simulink model "modal_closed_loop_control_Q27"  (R2025b)
settings: Solver=VariableStepAuto  StartTime=0.0  StopTime=200  RelTol=1e-3
undefined symbols (not defined in the file or in its folder): alpha, Den, eta_0, H, Jr, Js, K, Num, omega, sigma_m_square, taue, taum, Tc_max, theta_ref_FV, Torque_disturbance, xi
libraries: simulink_extras x2
settings Model: Creator=flori  LastModifiedBy=flori
settings DebuggingCC: AlgebraicLoopMsg=none

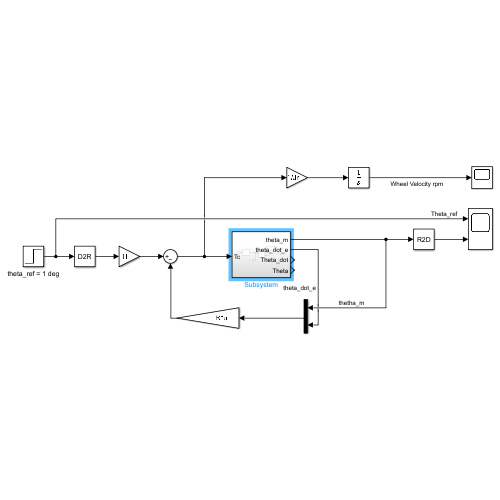
[thumbnail: Simulink's stored preview of the top-level diagram]
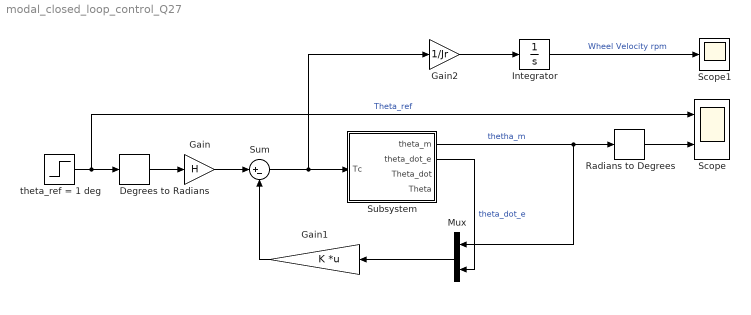
== system modal_closed_loop_control_Q27 ==
  Degrees to Radians : simulink_extras/Transformations/Degrees to Radians
  Gain : Gain  Gain=H
  Gain1 : Gain  Gain=K  Multiplication=Matrix(K*u)
  Gain2 : Gain  Gain=1/Jr
  Integrator : Integrator
  Mux : Mux  Inputs=2
  Radians to Degrees : simulink_extras/Transformations/Radians to Degrees
  Scope : Scope  NumInputPorts=2
      settings: ActiveDisplayYMinimum=-1.2780559634546143  ActiveDisplayYMaximum=11.460603856286715
  Scope1 : Scope
      settings: ActiveDisplayYMinimum=-162.46244989457873  ActiveDisplayYMaximum=1462.1620490512087
  Subsystem : Subsystem
  Sum : Sum  Inputs=|+-
  theta_ref = 1 deg : Step  Time=0  After=theta_ref_FV  SampleTime=0
  wires:
  Gain/1 -> Sum/1
  Mux/1 -> Gain1/1
  Subsystem/1(theta_m) -> Radians to Degrees/1, Mux/1  "thetha_m"
  Subsystem/2(theta_dot_e) -> Mux/2  "theta_dot_e"
  Gain2/1 -> Integrator/1
  Integrator/1 -> Scope1/1  "Wheel Velocity rpm"
  theta_ref = 1 deg/1 -> Scope/1, Degrees to Radians/1  "Theta_ref"
  Degrees to Radians/1 -> Gain/1
  Radians to Degrees/1 -> Scope/2
  Gain1/1 -> Sum/2
  Sum/1 -> Gain2/1, Subsystem/1(Tc)

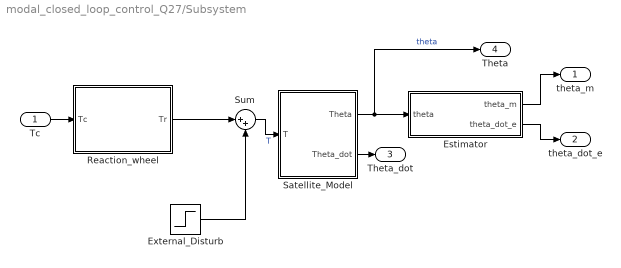
== system modal_closed_loop_control_Q27/Subsystem ==
  Tc : Inport
  Estimator : Subsystem
  External_Disturb : Step  Time=100  After=Torque_disturbance  SampleTime=0
  Reaction_wheel : Subsystem
  Satellite_Model : Subsystem
  Sum : Sum  Inputs=|++
  theta_m : Outport
  theta_dot_e : Outport  Port=2
  Theta_dot : Outport  Port=3
  Theta : Outport  Port=4
  wires:
  Satellite_Model/1(Theta) -> Theta/1, Estimator/1(theta)  "theta"
  Sum/1 -> Satellite_Model/1(T)  "T"
  Reaction_wheel/1(Tr) -> Sum/1
  Estimator/2(theta_dot_e) -> theta_dot_e/1
  Estimator/1(theta_m) -> theta_m/1
  Satellite_Model/2(Theta_dot) -> Theta_dot/1
  Tc/1 -> Reaction_wheel/1(Tc)
  External_Disturb/1 -> Sum/2

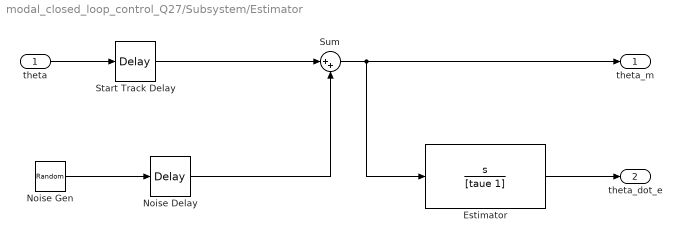
== system modal_closed_loop_control_Q27/Subsystem/Estimator ==
  theta : Inport
  Estimator : TransferFcn  Numerator=[1 0]  Denominator=[taue 1]
  Noise Delay : TransportDelay  DelayTime=160
  Noise Gen : RandomNumber  Variance=sigma_m_square  SampleTime=0.01
  Start Track Delay : TransportDelay  DelayTime=taum
  Sum : Sum  Inputs=|++
  theta_m : Outport
  theta_dot_e : Outport  Port=2
  wires:
  Start Track Delay/1 -> Sum/1
  Sum/1 -> theta_m/1, Estimator/1
  theta/1 -> Start Track Delay/1
  Estimator/1 -> theta_dot_e/1
  Noise Gen/1 -> Noise Delay/1
  Noise Delay/1 -> Sum/2

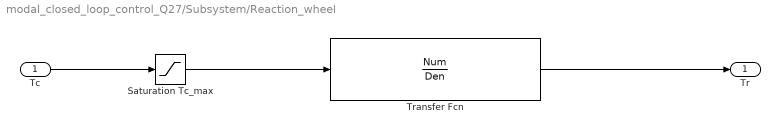
== system modal_closed_loop_control_Q27/Subsystem/Reaction_wheel ==
  Tc : Inport
  Saturation Tc_max : Saturate  UpperLimit=Tc_max  LowerLimit=-Tc_max
  Transfer Fcn : TransferFcn  Numerator=Num  Denominator=Den
  Tr : Outport
  wires:
  Transfer Fcn/1 -> Tr/1
  Saturation Tc_max/1 -> Transfer Fcn/1
  Tc/1 -> Saturation Tc_max/1

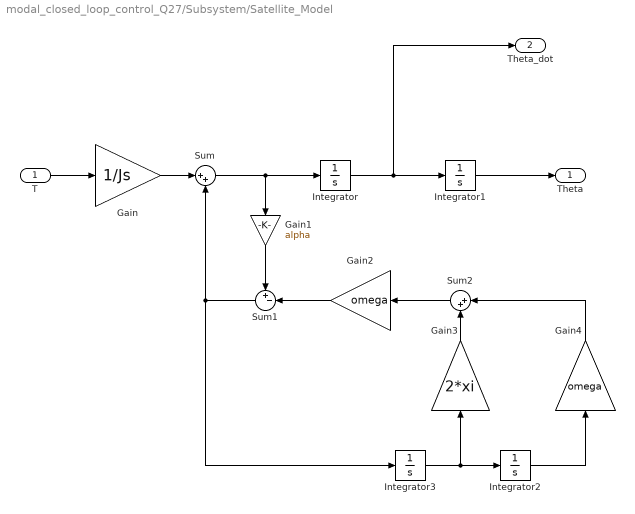
== system modal_closed_loop_control_Q27/Subsystem/Satellite_Model ==
  T : Inport
  Gain : Gain  Gain=1/Js
  Gain1 : Gain  Gain=alpha
  Gain2 : Gain  Gain=omega
  Gain3 : Gain  Gain=2*xi
  Gain4 : Gain  Gain=omega
  Integrator : Integrator
  Integrator1 : Integrator
  Integrator2 : Integrator  InitialCondition=eta_0
  Integrator3 : Integrator
  Sum : Sum  Inputs=|++
  Sum1 : Sum  Inputs=+-|
  Sum2 : Sum  Inputs=|++
  Theta : Outport
  Theta_dot : Outport  Port=2
  wires:
  Integrator/1 -> Theta_dot/1, Integrator1/1
  Gain4/1 -> Sum2/1
  Sum/1 -> Gain1/1, Integrator/1
  Gain2/1 -> Sum1/2
  Sum1/1 -> Integrator3/1, Sum/2
  Gain1/1 -> Sum1/1
  Gain3/1 -> Sum2/2
  Integrator3/1 -> Integrator2/1, Gain3/1
  Sum2/1 -> Gain2/1
  T/1 -> Gain/1
  Integrator1/1 -> Theta/1
  Gain/1 -> Sum/1
  Integrator2/1 -> Gain4/1
